simulink model "CLIK_con_pseudoinversa"  (R2022b)
settings: Solver=VariableStepAuto  StartTime=0.0  StopTime=40  RelTol=1e-3
values from neighbouring files (symbols this model uses):
  k_pinv = 10    [CLIK_script.m]
  T = T_A * T_B    [DH_dinamica.m]    (also in traiettoria_script.m = 0.001)
  theta1_0 = pi/2 - angolo    [CLIK_script.m]
  theta2_0 = 2*angolo    [CLIK_script.m]
undefined symbols (not defined in the file or in its folder): DiscIntNeverNeededParam
libraries: simulink x1
settings Model: Creator=Michele  LastModifiedBy=Michele
settings DataIOCC: ReturnWorkspaceOutputs=off

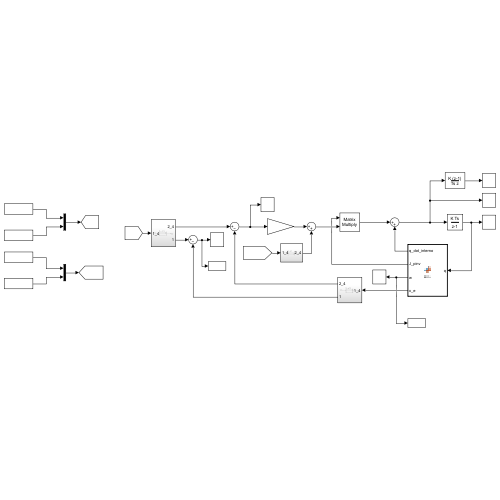
[thumbnail: Simulink's stored preview of the top-level diagram]
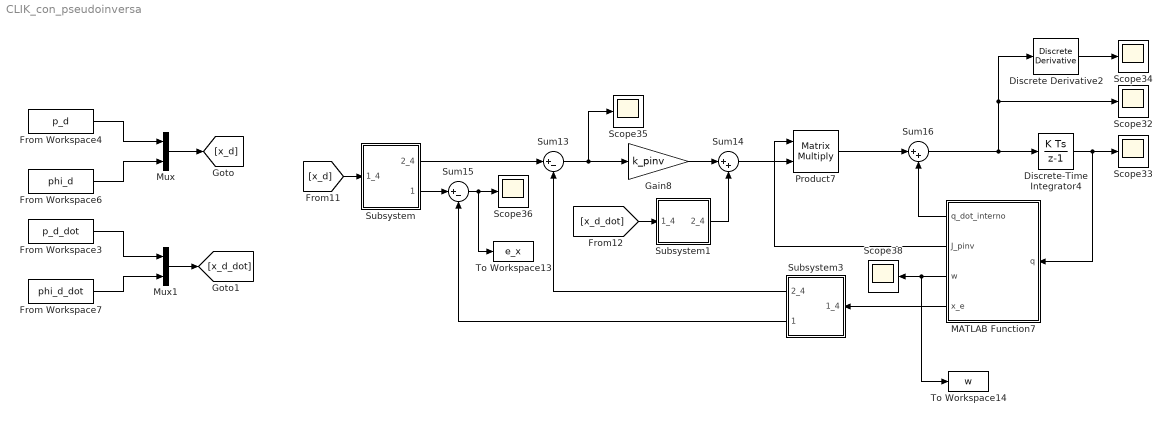
== system CLIK_con_pseudoinversa ==
  Discrete Derivative2 : simulink/Discrete/Discrete Derivative  gainval=1.0  ICPrevScaledInput=[0 0 0 0]'  OutMin=[]  OutMax=[]  OutDataType=fixdt(1, 16)  OutScaling=2^-10  DoSatur=off
  Discrete-Time Integrator4 : DiscreteIntegrator  InitialCondition=[theta1_0 theta2_0 -0.25 0]'  SampleTime=-1  ICPrevOutput=DiscIntNeverNeededParam  ICPrevScaledInput=DiscIntNeverNeededParam
  From Workspace3 : FromWorkspace  VariableName=p_d_dot  SampleTime=T
  From Workspace4 : FromWorkspace  VariableName=p_d  SampleTime=T
  From Workspace6 : FromWorkspace  VariableName=phi_d  SampleTime=T
  From Workspace7 : FromWorkspace  VariableName=phi_d_dot  SampleTime=T
  Gain8 : Gain  Gain=k_pinv
  MATLAB Function7 : MATLAB Function  TreatAsAtomicUnit=on
  Mux : Mux  Inputs=2
  Mux1 : Mux  Inputs=2
  Product7 : Product  Multiplication=Matrix(*)
  Scope{32..36,38} (6 alike) : Scope
  Subsystem : Subsystem
  Subsystem1 : Subsystem
  Subsystem3 : Subsystem
  Sum13 : Sum  Inputs=|+-
  Sum14 : Sum  Inputs=|++
  Sum15 : Sum  Inputs=|+-
  Sum16 : Sum  Inputs=|++
  To Workspace13 : ToWorkspace  VariableName=e_x  SaveFormat=Structure With Time  SampleTime=-1
  To Workspace14 : ToWorkspace  VariableName=w  SaveFormat=Structure With Time  SampleTime=-1
  wires:
  Gain8/1 -> Sum14/1
  Sum16/1 -> Discrete Derivative2/1, Scope32/1, Discrete-Time Integrator4/1
  Discrete Derivative2/1 -> Scope34/1
  MATLAB Function7/3(w) -> To Workspace14/1, Scope38/1
  Product7/1 -> Sum16/1
  MATLAB Function7/2(J_pinv) -> Product7/1
  Sum13/1 -> Gain8/1, Scope35/1
  Discrete-Time Integrator4/1 -> MATLAB Function7/1(q), Scope33/1
  MATLAB Function7/1(q_dot_interno) -> Sum16/2
  [x_d] -> Subsystem/1(1_4)
  Subsystem/1(2_4) -> Sum13/1
  MATLAB Function7/4(x_e) -> Subsystem3/1(1_4)
  [x_d_dot] -> Subsystem1/1(1_4)
  Sum14/1 -> Product7/2
  Subsystem1/1(2_4) -> Sum14/2
  Subsystem/2(1) -> Sum15/1
  Sum15/1 -> To Workspace13/1, Scope36/1
  Subsystem3/1(2_4) -> Sum13/2
  Subsystem3/2(1) -> Sum15/2
  Mux1/1 -> [x_d_dot]
  From Workspace3/1 -> Mux1/1
  Mux/1 -> [x_d]
  From Workspace7/1 -> Mux1/2
  From Workspace4/1 -> Mux/1
  From Workspace6/1 -> Mux/2

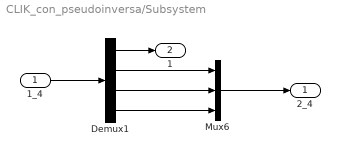
== system CLIK_con_pseudoinversa/Subsystem ==
  1_4 : Inport
  Demux1 : Demux
  Mux6 : Mux  Inputs=3
  2_4 : Outport
  1 : Outport  Port=2
  wires:
  Mux6/1 -> 2_4/1
  Demux1/4 -> Mux6/3
  1_4/1 -> Demux1/1
  Demux1/2 -> Mux6/1
  Demux1/3 -> Mux6/2
  Demux1/1 -> 1/1

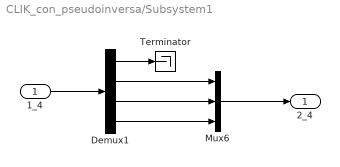
== system CLIK_con_pseudoinversa/Subsystem1 ==
  1_4 : Inport
  Demux1 : Demux
  Mux6 : Mux  Inputs=3
  Terminator : Terminator
  2_4 : Outport
  wires:
  Mux6/1 -> 2_4/1
  Demux1/4 -> Mux6/3
  1_4/1 -> Demux1/1
  Demux1/2 -> Mux6/1
  Demux1/3 -> Mux6/2
  Demux1/1 -> Terminator/1

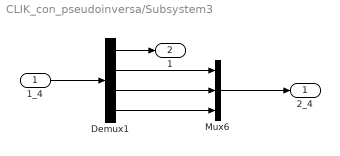
== system CLIK_con_pseudoinversa/Subsystem3 ==
  1_4 : Inport
  Demux1 : Demux
  Mux6 : Mux  Inputs=3
  2_4 : Outport
  1 : Outport  Port=2
  wires:
  Mux6/1 -> 2_4/1
  Demux1/4 -> Mux6/3
  1_4/1 -> Demux1/1
  Demux1/2 -> Mux6/1
  Demux1/3 -> Mux6/2
  Demux1/1 -> 1/1

== matlab function CLIK_con_pseudoinversa/MATLAB Function7 ==
  data: q_dot_interno output; J_pinv output; w output; q input; x_e output
function [q_dot_interno,J_pinv,w,x_e] = kin(q)

    q1 = q(1); q2 = q(2); q3 = q(3); q4 = q(4);

    J = [- sin(q1)/2 - (cos(q1)*sin(q2))/2 - (cos(q2)*sin(q1))/2, - (cos(q1)*sin(q2))/2 - (cos(q2)*sin(q1))/2, 0, 0;
           cos(q1)/2 + (cos(q1)*cos(q2))/2 - (sin(q1)*sin(q2))/2,   (cos(q1)*cos(q2))/2 - (sin(q1)*sin(q2))/2, 0, 0;
                                                               0,                                           0, 1, 0;
                                                               0,                                           0, 0, 1];

    x_e = [cos(q1)/2 + (cos(q1)*cos(q2))/2 - (sin(q1)*sin(q2))/2;
           sin(q1)/2 + (cos(q1)*sin(q2))/2 + (cos(q2)*sin(q1))/2;
                                                   q3;
                                                   q4];
    J = J(2:end,:);

    J_pinv = pinv(J);

    P = eye(4) - J_pinv*J;
    q_dot_interno = P * 5 * [0 cos(q(2)) 0 0]';

    w = sqrt(det(J*J'));
end
